simulink model "Model_MotorDC_14b"  (R2014b)
settings: Solver=ode45  StartTime=0.0  StopTime=10  RelTol=1e-3
undefined symbols (not defined in the file or in its folder): in
settings Model: Creator=Zer0  LastModifiedBy=Arek

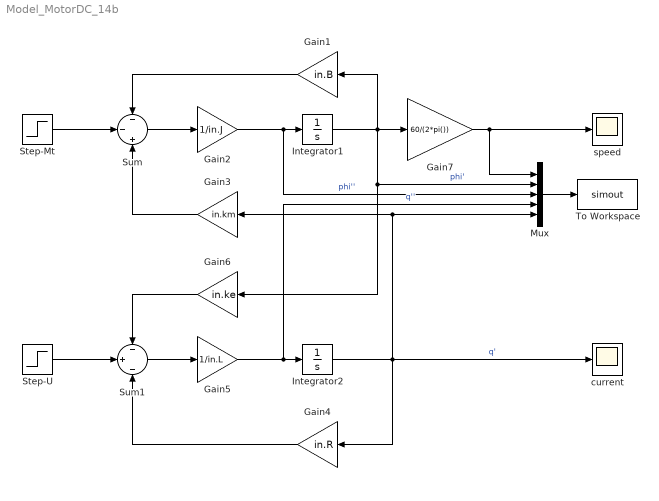
== system Model_MotorDC_14b ==
  Gain1 : Gain  Gain=in.B
  Gain2 : Gain  Gain=1/in.J
  Gain3 : Gain  Gain=in.km
  Gain4 : Gain  Gain=in.R
  Gain5 : Gain  Gain=1/in.L
  Gain6 : Gain  Gain=in.ke
  Gain7 : Gain  Gain=60/(2*pi())
  Integrator1 : Integrator
  Integrator2 : Integrator
  Mux : Mux  Inputs=5
  Step-Mt : Step  Time=2  After=in.Mt  SampleTime=0
  Step-U : Step  After=in.U  SampleTime=0
  Sum : Sum  Inputs=-|-|+
  Sum1 : Sum  Inputs=-|+|-
  To Workspace : ToWorkspace  VariableName=simout  SaveFormat=Timeseries  SampleTime=-1
  current : Scope
      settings: YMin=-1  YMax=1
  speed : Scope
      settings: TimeRange=1.2  YMin=-1  YMax=1
  wires:
  Mux/1 -> To Workspace/1
  Integrator1/1 -> Gain7/1, Gain1/1, Gain6/1, Mux/2  "phi'"
  Gain2/1 -> Mux/3, Integrator1/1  "phi''"
  Sum/1 -> Gain2/1
  Gain1/1 -> Sum/1
  Step-Mt/1 -> Sum/2
  Gain3/1 -> Sum/3
  Gain5/1 -> Mux/4, Integrator2/1  "q''"
  Integrator2/1 -> current/1, Gain4/1, Mux/5, Gain3/1  "q'"
  Gain4/1 -> Sum1/3
  Sum1/1 -> Gain5/1
  Gain6/1 -> Sum1/1
  Step-U/1 -> Sum1/2
  Gain7/1 -> Mux/1, speed/1
